simulink model "Sinusoidal_PWM"  (R2023b)
settings: Solver=VariableStepAuto  StartTime=0.0  StopTime=1.0  MaxStep=1e-5  RelTol=1e-3
undefined symbols (not defined in the file): fs
libraries: simulink x1
settings Model: Creator=HP  LastModifiedBy=HP

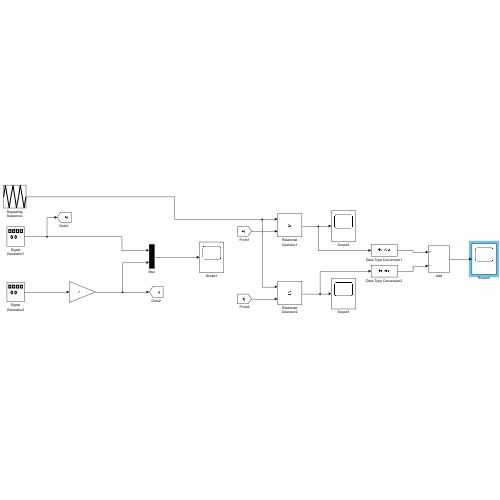
[thumbnail: Simulink's stored preview of the top-level diagram]
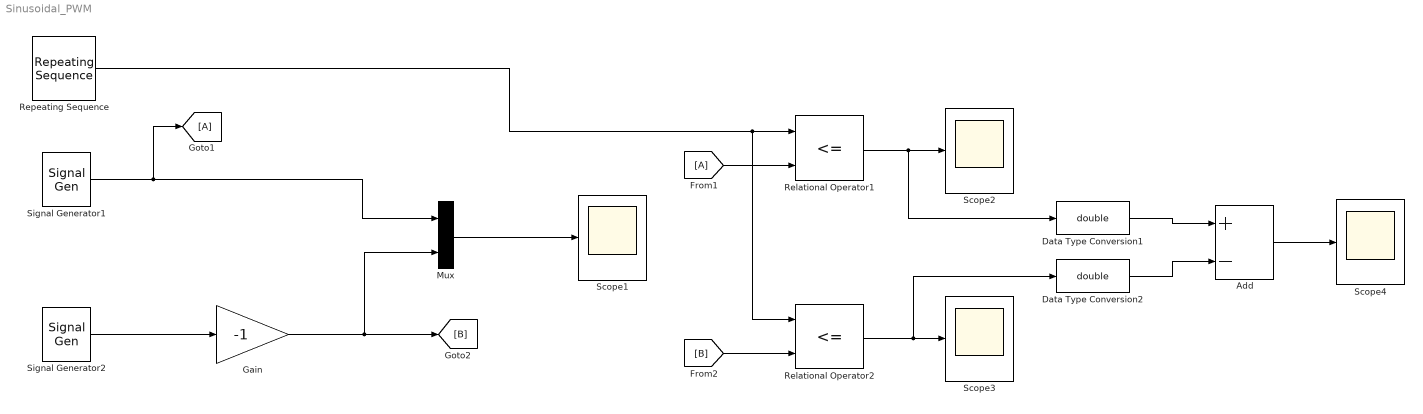
== system Sinusoidal_PWM ==
  Add : Sum  Inputs=+-
  Data Type Conversion1 : DataTypeConversion  OutDataTypeStr=double  SaturateOnIntegerOverflow=off  RndMeth=Floor
  Data Type Conversion2 : DataTypeConversion  OutDataTypeStr=double  SaturateOnIntegerOverflow=off  RndMeth=Floor
  From1 : From
  Gain : Gain  Gain=-1
  Goto1 : Goto
  Mux : Mux  Inputs=2
  Relational Operator1 : RelationalOperator  Operator=<=  OutDataTypeStr=boolean  RndMeth=Simplest  InputSameDT=off
  Relational Operator2 : RelationalOperator  Operator=<=  OutDataTypeStr=boolean  RndMeth=Simplest  InputSameDT=off
  Repeating Sequence : simulink/Sources/Repeating Sequence  rep_seq_t=[0 1/fs/4 3/fs/4 1/fs]  rep_seq_y=[0 1 -1 0]
  Scope{1..4} (4 alike) : Scope
  Signal Generator1 : SignalGenerator  Frequency=60
  Signal Generator2 : SignalGenerator  Frequency=60
  wires:
  Signal Generator2/1 -> Gain/1
  Gain/1 -> [B], Mux/2
  Signal Generator1/1 -> Goto1/1, Mux/1
  Mux/1 -> Scope1/1
  From1/1 -> Relational Operator1/2
  Repeating Sequence/1 -> Relational Operator2/1, Relational Operator1/1
  Relational Operator1/1 -> Data Type Conversion1/1, Scope2/1
  [B] -> Relational Operator2/2
  Relational Operator2/1 -> Data Type Conversion2/1, Scope3/1
  Add/1 -> Scope4/1
  Data Type Conversion1/1 -> Add/1
  Data Type Conversion2/1 -> Add/2
